simulink model "HighDegNonLinSystem"  (R2025b)
settings: Solver=VariableStepAuto  StartTime=0.0  StopTime=20  RelTol=1e-3
values from neighbouring files (symbols this model uses):
  hiddenLayerSizeCtrl = 20    [Init.m]
  hiddenLayerSizeObsv = 5    [Init.m]
  n = 2    [Init.m]
  p = 1    [Init.m]
  u_max = 5    [Init.m]
  u_min = - 5    (= -5)    [Init.m]
  Vctrl0 = 0.1 * randn(hiddenLayerSizeCtrl, inputLayerSizeCtrl)    [Init.m]
  Vobsv0 = 0.1 * randn(hiddenLayerSizeObsv, inputLayerSizeObsv)    [Init.m]
  Wctrl0 = 0.1 * randn(outputLayerSizeCtrl, hiddenLayerSizeCtrl)    [Init.m]
  Wobsv0 = 0.1 * randn(outputLayerSizeObsv, hiddenLayerSizeObsv)    [Init.m]
  x0 = [0.5; 0.5]    [Init.m]
  x_hat0 = [1; 0]    [Init.m]
settings Model: Creator=Asus  LastModifiedBy=Asus

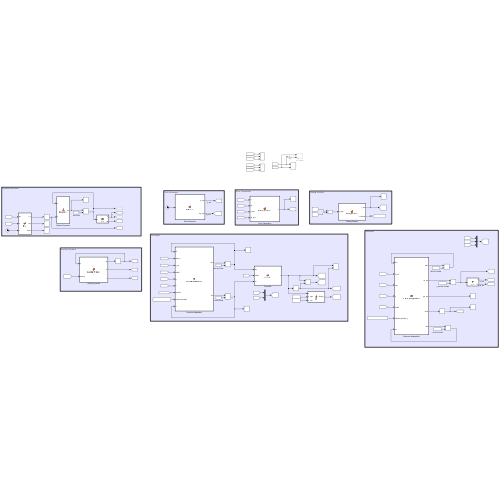
[thumbnail: Simulink's stored preview of the top-level diagram]
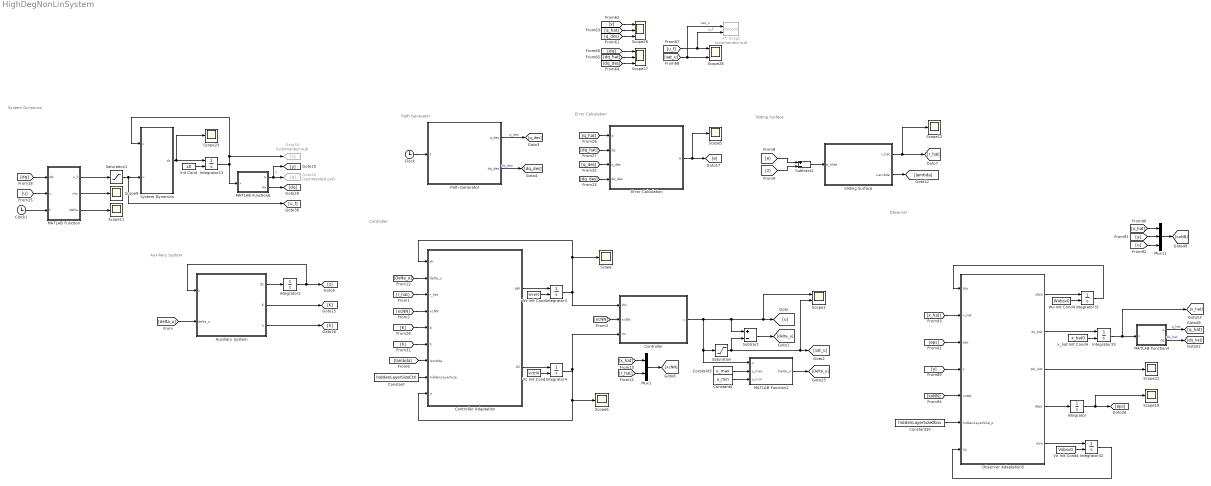
== system HighDegNonLinSystem ==
  note: Path Generator
  note: Auxiliary System
  note: Controller
  note: Sliding Surface
  note: Error Calculation
  note: Observer
  note: System Dynamics
  Auxiliary System : MATLAB Function  TreatAsAtomicUnit=on
  Clock : Clock
  Clock1 : Clock
  Constant : Constant  Value=hiddenLayerSizeCtrl
  Constant10 : Constant  Value=hiddenLayerSizeObsv
  Constant3 : Constant  Value=u_max
  Constant4 : Constant  Value=u_min
  Controller : MATLAB Function  TreatAsAtomicUnit=on
  Controller Adaptation : MATLAB Function  TreatAsAtomicUnit=on
  Error Calculation : MATLAB Function  TreatAsAtomicUnit=on
  Goto28 : Goto  Commented=on  GotoTag=q
  Goto30 : Goto  Commented=on  GotoTag=x
  Init Cond : Constant  Value=x0
  Integrator : Integrator  InitialCondition=1 * ones(p, 1)
  Integrator{3..4,13,31..33} (6 alike) : Integrator  InitialConditionSource=external  InitialCondition=[0.5; 0.5]
  Integrator2 : Integrator  InitialCondition=zeros(n, 1)
  MATLAB Function : MATLAB Function  TreatAsAtomicUnit=on
  MATLAB Function2 : MATLAB Function  TreatAsAtomicUnit=on
  MATLAB Function4 : MATLAB Function  TreatAsAtomicUnit=on
  MATLAB Function6 : MATLAB Function  TreatAsAtomicUnit=on
  Mux1 : Mux  Inputs=2
  Mux11 : Mux  Inputs=3
  Observer Adaptation5 : MATLAB Function  TreatAsAtomicUnit=on
  Path Generator : MATLAB Function  TreatAsAtomicUnit=on
  Saturation : Saturate  UpperLimit=u_max  LowerLimit=u_min
  Saturation1 : Saturate  UpperLimit=u_max  LowerLimit=u_min
  Scope{,5..6,9,11..12,19,22..23} (9 alike) : Scope
      Scope settings: ActiveDisplayYMinimum=-0.80632877657571234  ActiveDisplayYMaximum=0.81297662531396131
      Scope11 settings: ActiveDisplayYMinimum=-1  ActiveDisplayYMaximum=1  DataLoggingVariableName=ScopeData6
      Scope12 settings: ActiveDisplayYMinimum=-7.8844362962481993  ActiveDisplayYMaximum=3.2414659891040802  DataLoggingVariableName=ScopeData7
      Scope19 settings: ActiveDisplayYMinimum=-3.0403147891291562  ActiveDisplayYMaximum=37.362833102162412  DataLoggingVariableName=ScopeData15
      Scope22 settings: ActiveDisplayYMinimum=-1  ActiveDisplayYMaximum=1  DataLoggingVariableName=ScopeData18
      Scope23 settings: ActiveDisplayYMinimum=-17.129349977314451  ActiveDisplayYMaximum=21.988712096819278  DataLoggingVariableName=ScopeData19
      Scope5 settings: ActiveDisplayYMinimum=-0.20021441252280484  ActiveDisplayYMaximum=0.22401805193004884
      Scope6 settings: ActiveDisplayYMinimum=-1  ActiveDisplayYMaximum=1  DataLoggingVariableName=ScopeData2
      Scope9 settings: ActiveDisplayYMinimum=0.80707640666393865  ActiveDisplayYMaximum=1.1881026214817845  DataLoggingVariableName=ScopeData5
  Scope1 : Scope  NumInputPorts=2
      settings: ActiveDisplayYMinimum=-6.1356708767818073  ActiveDisplayYMaximum=5.2210378910362634  DataLoggingVariableName=ScopeData3
  Scope26 : Scope  NumInputPorts=3
      settings: ActiveDisplayYMinimum=-1.0151291113135565  ActiveDisplayYMaximum=1.2239032345903951  DataLoggingVariableName=ScopeData22
  Scope27 : Scope  NumInputPorts=3
      settings: ActiveDisplayYMinimum=-27.452996869718429  ActiveDisplayYMaximum=14.646456806157516  DataLoggingVariableName=ScopeData23
  Scope28 : Scope  NumInputPorts=2
      settings: ActiveDisplayYMinimum=-6.1356708767818073  ActiveDisplayYMaximum=5.2210378910362634  DataLoggingVariableName=ScopeData24
  Sliding Surface : MATLAB Function  TreatAsAtomicUnit=on
  Subtract : Sum  Inputs=+-
  Subtract1 : Sum  Inputs=+-
  System Dynamics : MATLAB Function  TreatAsAtomicUnit=on
  Vc Init Cond : Constant  Value=Vctrl0
  Vo Init Cond4 : Constant  Value=Vobsv0
  Wc Init Cond : Constant  Value=Wctrl0
  Wo Init Cond4 : Constant  Value=Wobsv0
  XY Graph : Record  Commented=on  NumPorts=2.0  FileSettingsInternal="{\"entries\":[{\"content\":{\"excelSettings\":{\"content\":{},\"type\":\"Streamout.ExcelSettings\"},\"parquetSettings\":{\"content\":{},\"type\":\"Streamout.ParquetSettings\"}},\"type\":\"Streamout.FileSettingStorage\",\"uuid\":\"\"}],\"packageUris\":[\"http:\\/\\/schema.mathworks.com\\/mf0\\/streamout_blocks\\/R2020a\"],\"version\":\"1.0\"}"  FrameSettings=[0, 0]  Layout=[1 1]  SignalsInternal="{\"entries\":[{\"content\":{\"signals\":[{\"content\":{\"blockPath\":[],\"dimensions\":[3,1],\"domain\":\"\",\"hasChildren\":true,\"lineColor\":\"#64d413\",\"lineWidth\":2,\"port\":1,\"signalID\":1,\"signalName\":\"sat_u\"},\"type\":\"RecordBlkView.Signal\",\"uuid\":\"\"},{\"content\":{\"blockPath\":[],\"channel\":[1,1],\"dimensions\":[3,1],\"domain\":\"\",\"lineColor\":\"#7e2f8e\",\"lineWidth\":2,\"parentID\":1,\"port\":1,\"signalID\":2,\"signalName\":\"sat_u\"},\"type\":\"RecordBlkView.Signal\",\"uuid\":\"\"},{\"content\":{\"blockPath\":[],\"channel\":[2,1],\"dimensions\":[3,1],\"domain\":\"\",\"lineColor\":\"#a2142f\",\"lineWidth\":2,\"parentID\":1,\"plots\":[ 1 ],\"port\":1,\"signalID\":3,\"signalName\":\"sat_u\"},\"type\":\"RecordBlkView.Signal\",\"uuid\":\"\"},{\"content\":{\"blockPath\":[],\"channel\":[3,1],\"dimensions\":[3,1],\"domain\":\"\",\"lineColor\":\"#139fff\",\"lineWidth\":2,\"parentID\":1,\"port\":1,\"signalID\":4,\"signalName\":\"sat_u\"},\"type\":\"RecordBlkView.Signal\",\"uuid\":\"\"},{\"content\":{\"blockPath\":[],\"dimensions\":[3,1],\"domain\":\"\",\"hasChildren\":true,\"lineColor\":\"#fe330a\",\"lineWidth\":2,\"port\":2,\"signalID\":5,\"signalName\":\"u_f\"},\"type\":\"RecordBlkView.Signal\",\"uuid\":\"\"},{\"content\":{\"blockPath\":[],\"channel\":[1,1],\"dimensions\":[3,1],\"domain\":\"\",\"lineColor\":\"#4dbeee\",\"lineWidth\":2,\"parentID\":5,\"port\":2,\"signalID\":6,\"signalName\":\"u_f\"},\"type\":\"RecordBlkView.Signal\",\"uuid\":\"\"},{\"content\":{\"blockPath\":[],\"channel\":[2,1],\"dimensions\":[3,1],\"domain\":\"\",\"lineColor\":\"#ff6929\",\"lineWidth\":2,\"parentID\":5,\"plots\":[ 1 ],\"port\":2,\"signalID\":7,\"signalName\":\"u_f\"},\"type\":\"RecordBlkView.Signal\",\"uuid\":\"\"},{\"content\":{\"blockPath\":[],\"channel\":[3,1],\"dimensions\":[3,1],\"domain\":\"\",\"lineColor\":\"#b746ff\",\"lineWidth\":2,\"parentID\":5,\"port\":2,\"signalID\":8,\"signalName\":\"u_f\"},\"type\":\"RecordBlkView.Signal\",\"uuid\":\"\"}]},\"type\":\"RecordBlkView.InputSignals\",\"uuid\":\"\"}],\"packageUris\":[\"http:\\/\\/schema.mathworks.com\\/mf0\\/streamout_blocks\\/R2020a\"],\"version\":\"1.0\"}"  VisualizationBindings="{\"xyplotplugin\":{\"info\":[{\"series\":[{\"bindingParametersList\":[{\"parameter\":\"X-Axis\",\"signalID\":3,\"signalName\":\"sat_u(2,1)\"},{\"parameter\":\"Y-Axis\",\"signalID\":7,\"signalName\":\"u_f(2,1)\"}],\"seriesID\":0}],\"subplotID\":1}]}}"  CompatibilityTag=XY
  x_hat Init Cond4 : Constant  Value=x_hat0
  wires:
  Clock/1 -> Path Generator/1(t)
  Auxiliary System/1(dz) -> Integrator2/1
  Integrator2/1 -> [z], Auxiliary System/1(z)
  Controller/1(u) -> Scope1/1, [u], Subtract/1, MATLAB Function2/1(u), Saturation/1
  Wc Init Cond/1 -> Integrator3/2
  Controller Adaptation/1(dW) -> Integrator3/1
  Integrator3/1 -> Controller/1(Wc), Scope/1, Controller Adaptation/1(W)
  Controller Adaptation/2(dV) -> Integrator4/1
  Vc Init Cond/1 -> Integrator4/2
  Integrator4/1 -> Controller/3(Vc), Scope6/1, Controller Adaptation/9(V)
  [r_hat] -> Controller Adaptation/3(r_hat)
  [xcNN] -> Controller Adaptation/4(xcNN)
  [xcNN] -> Controller/2(xcNN)
  Mux1/1 -> [xcNN]
  [r_hat] -> Mux1/2
  Saturation/1 -> Scope1/2, [sat_u], Subtract/2
  [Delta_u] -> Controller Adaptation/2(delta_u)
  Constant/1 -> Controller Adaptation/8(hiddenLayerSize)
  Sliding Surface/1(r_hat) -> Scope12/1, [r_hat]
  Path Generator/2(dq_des) -> [dq_des]  "dq_des"
  Path Generator/1(q_des) -> [q_des]  "q_des"
  [lambda] -> Controller Adaptation/7(lambda)
  Sliding Surface/2(Lambda) -> [lambda]
  Error Calculation/1(e) -> Scope5/1, [e]
  [q_des] -> Error Calculation/3(q_des)
  [dq_des] -> Error Calculation/4(dq_des)
  [x_hat] -> Mux1/1
  [delta_u] -> Auxiliary System/2(delta_u)
  Subtract/1 -> [delta_u]
  [dq_hat] -> Error Calculation/2(dq)
  Observer Adaptation5/2(dx_hat) -> Integrator33/1
  Observer Adaptation5/5(dVo) -> Integrator32/1
  Mux11/1 -> [xoNN]
  MATLAB Function4/2(dq) -> [dq_hat]  "dq_hat"
  [xoNN] -> Observer Adaptation5/5(xoNN)
  Integrator32/1 -> Observer Adaptation5/7(Vo)
  MATLAB Function4/1(q) -> [q_hat]  "q_hat"
  [u] -> Mux11/3
  [y] -> Observer Adaptation5/4(y)
  Wo Init Cond4/1 -> Integrator31/2
  Constant10/1 -> Observer Adaptation5/6(hiddenLayerSize_o)
  [x_hat] -> Observer Adaptation5/2(x_hat)
  Integrator31/1 -> Observer Adaptation5/1(Wo)
  x_hat Init Cond4/1 -> Integrator33/2
  [x_hat] -> Mux11/1
  Vo Init Cond4/1 -> Integrator32/2
  [y] -> Mux11/2
  [q_hat] -> Error Calculation/1(q)
  MATLAB Function6/1(q) -> [y], Goto28/1  "y"
  Integrator13/1 -> System Dynamics/1(x), Goto30/1, MATLAB Function6/1(x)
  System Dynamics/1(dx) -> Scope23/1, Integrator13/1
  MATLAB Function6/2(dq) -> [dq]
  Init Cond/1 -> Integrator13/2
  Observer Adaptation5/1(dWo) -> Integrator31/1
  MATLAB Function2/1(Delta_u) -> [Delta_u]
  Constant3/1 -> MATLAB Function2/2(u_max)
  Constant4/1 -> MATLAB Function2/3(u_min)
  Integrator33/1 -> MATLAB Function4/1(x), [x_hat]
  Observer Adaptation5/4(deps) -> Integrator/1
  Integrator/1 -> Scope19/1, [eps]
  [eps] -> Observer Adaptation5/3(eps)
  Observer Adaptation5/3(psi_hat) -> Scope22/1
  [e] -> Subtract1/1
  Subtract1/1 -> Sliding Surface/1(e_tilde)
  [z] -> Subtract1/2
  [y] -> Scope26/1
  [q_hat] -> Scope26/2
  [q_des] -> Scope26/3
  [dq] -> Scope27/1
  [dq_hat] -> Scope27/2
  [dq_des] -> Scope27/3
  Saturation1/1 -> [u_f], System Dynamics/2(u)
  [u_f] -> XY Graph/2, Scope28/1  "u_f"
  [sat_u] -> XY Graph/1, Scope28/2  "sat_u"
  Clock1/1 -> MATLAB Function/3(t)
  MATLAB Function/1(u_f) -> Saturation1/1
  [u] -> MATLAB Function/2(u)
  [dq] -> MATLAB Function/1(dq)
  MATLAB Function/2(rho) -> Scope9/1
  MATLAB Function/3(delta) -> Scope11/1
  [K] -> Controller Adaptation/5(K)
  [h] -> Controller Adaptation/6(h)
  Auxiliary System/2(K) -> [K]
  Auxiliary System/3(h) -> [h]

== matlab function HighDegNonLinSystem/Controller Adaptation ==
  data: dW output; dV output; W input; delta_u input; r_hat input; xcNN input; K input; h input; lambda input; hiddenLayerSize input; V input
function [dW, dV] = ControllerAdaptation(W, delta_u, r_hat, xcNN, K, h, lambda, hiddenLayerSize, V)
    
    Sigma = @(z) (-1 + 2 ./ (1 + exp(-2 * z)));
    Sigma_c  = Sigma(V * xcNN);

    l = 2;

    A = [0, 1; 0, 0];
    B = [0; 1];

    Ac = A - B * ([lambda', 1] * l + [0, lambda']);

    eta   = 10 * [0.1, 0.1];
    gamma = [0.001, 0.001];

    PI_c      = diag(Sigma_c.^2);
    PI_lambda = [lambda', 1];
    
    dW = eta(1) * (r_hat' * PI_lambda * (-Ac^(-1) * B + K^(-1) * h * diag(delta_u)))' * Sigma_c' - gamma(1) * norm(r_hat) * W';
    dV = eta(2) * (r_hat' * PI_lambda * (-Ac^(-1) * B + K^(-1) * h * diag(delta_u)) * W' * (eye(hiddenLayerSize) - PI_c))' * xcNN' - gamma(2) * norm(r_hat) * V;

end

== matlab function HighDegNonLinSystem/Sliding Surface ==
  data: e_tilde input; r_hat output; Lambda output
function [r_hat, Lambda] = SlidingSurface(e_tilde)

    Lambda = 10;

    r_hat = [Lambda, 1] * e_tilde;

end

== matlab function HighDegNonLinSystem/Error Calculation ==
  data: e output; q input; dq input; q_des input; dq_des input
function e = ErrorCalculation(q, dq, q_des, dq_des)

    y_bar = [q(1); dq(1)];
    y_bar_des = [q_des(1); dq_des(1)];
    e = y_bar - y_bar_des;
    
end

== matlab function HighDegNonLinSystem/MATLAB Function2 ==
  data: u input; Delta_u output; u_max input; u_min input
function Delta_u = fcn(u, u_max, u_min)

    if u > u_max
        Delta_u   = 1;
    elseif u < u_min
        Delta_u   = 1;
    else
        Delta_u   = 0;
    end

end

== matlab function HighDegNonLinSystem/MATLAB Function6 ==
  data: x input; q output; dq output
function [q, dq] = fcn(x)

    q  = x(1);
    dq = x(2);

end

== matlab function HighDegNonLinSystem/System Dynamics ==
  data: x input; dx output; u input
function dx = Dynamics(x, u)

    A = [0, 1; 0, 0];
    B = [0; 1];

    % dynamics
    psi = (x(1) + x(2)) / (1 + (x(1) + x(2))^2) ...
    + (1 + x(2)^2) * x(1)^2 + x(1) * cos(x(1)) * sin(x(2)) ...
    + 0.5 * sin(x(2) * exp(-x(1)^2)) + log(3 + cos(x(1)) ...
    + sin(x(1)*x(2))^2) - log(1 + x(1)^2*x(2)^2) ...
    + (2 + cos(x(1)*x(2))) * u + 0.1*u^3 + sin(0.5*u) + tanh(u);
    dx  = A * x + B * psi;

end

== matlab function HighDegNonLinSystem/MATLAB Function4 ==
  data: x input; q output; dq output
function [q, dq] = fcn(x)

    q  = x(1);
    dq = x(2);

end

== matlab function HighDegNonLinSystem/Observer Adaptation5 ==
  data: dWo output; dx_hat output; psi_hat output; deps output; dVo output; Wo input; x_hat input; eps input; y input; xoNN input; hiddenLayerSize_o input; Vo input
function [dWo, dx_hat, psi_hat, deps, dVo] = ObserverAdaptation(Wo, x_hat, eps, y, xoNN, hiddenLayerSize_o, Vo)

    Sigma = @(z) (-1 + 2 ./ (1 + exp(-2 * z)));
    Sigma_o = Sigma(Vo * xoNN);

    A = [0, 1; 0, 0];
    B = [0; 1];
    C = [1; 0];
    
    y_hat   = C' * x_hat;
    y_tilde = y - y_hat;

    alpha  = [2, 10];
    lambda = 0.01;
    kappa  = 100 ./ lambda;
    
    if abs(y_tilde) > lambda
        deps = kappa * y_tilde^2;
    else
        deps = 0;
    end
    
    rho = 2;
    Ho  = alpha(1, 2)*eps^rho;
    
    D = [alpha(1, 1)*eps; 0];
    
    Ao   = A  - D*C';
    Aocl = Ao - B*Ho*C';

    psi_hat = Wo' * Sigma_o;
    dx_hat  = Ao * x_hat + B * (psi_hat + Ho * y_tilde) + D * y;

    eta_o   = 5 * [10, 10];
    gamma_o = 1 * [0.01, 0.01];

    PI_o = diag(Sigma_o.^2);

    dWo = - eta_o(1) * (y_tilde' * C' * Aocl^(-1) * B)' * Sigma_o' - gamma_o(1) * norm(y_tilde) * Wo';
    dVo = - eta_o(2) * (y_tilde' * C' * Aocl^(-1) * B * Wo' * (eye(hiddenLayerSize_o) - PI_o))' * xoNN' - gamma_o(2) * norm(y_tilde) * Vo;

    % dWo = zeros(size(Wo));
    % dVo = zeros(size(Vo));

end

== matlab function HighDegNonLinSystem/Auxiliary System ==
  data: z input; dz output; delta_u input; K output; h output
function [dz, K, h] = AuxiliarySystem(z, delta_u)
    
    K = 5  * diag([-1, -1]);
    h = 0.05 * [-1; -1];

    dz = K * z + h .* delta_u;
    
end

== matlab function HighDegNonLinSystem/MATLAB Function ==
  data: dq input; u input; u_f output; t input; rho output; delta output
function [u_f, rho, delta] = fcn(dq, u, t)

    rho   = 0.70 + 0.30 * exp(-0.05 * t) - 0.1 * tanh(abs(dq) / 2);
    delta = -0.15 * tanh(dq) - 0.2 * dq;
    u_f   = rho .* u + delta;

end

== matlab function HighDegNonLinSystem/Path Generator ==
  data: t input; q_des output; dq_des output
function [q_des, dq_des] = PathGen(t)
    
    q_des   =   0.5 * cos(1.3 * t + pi/3) + 0.3 * sin(t);
    dq_des  = - 0.5 * 1.3 * sin(1.3 * t + pi/3) + 0.3 * cos(t);
    
end

== matlab function HighDegNonLinSystem/Controller ==
  data: u output; Wc input; xcNN input; Vc input
function u = Controller(Wc, xcNN, Vc)

    Sigma = @(z) (-1 + 2 ./ (1 + exp(-2 * z)));
    u = - Wc' * Sigma(Vc * xcNN);
    
end
